simulink model "LPV_ReducedLPV_Simulation_16b"  (R2016b)
settings: Solver=FixedStepAuto  StartTime=0.0  StopTime=10  FixedStep=ts  RelTol=1e-3
values from neighbouring files (symbols this model uses):
  Im = (1/m)*ones(m,m)    [KPCA_Gaussian.m]    (also in KPCA_Polynomial.m)
  ITest = (1/m)*ones(1,m)    [Reduced_LPV_System.m]
  Kernel_Var = 100    [KPCA_Gaussian.m]    (also in KPCA_Polynomial.m = 2)
  KernelMatrix = zeros(m,m)    [KPCA_Gaussian.m]    (also in KPCA_Polynomial.m)
  KTest = zeros(1,m)    [Reduced_LPV_System.m]
  l = 5    [KPCA_Gaussian.m]    (also in KPCA_Polynomial.m; Plot_Accuracy_Gaussian.m = 6; Plot_Accuracy_PCA_Polynomial.m = 6; Plot_Accuracy_Polynomial.m = 6)
  m = 7000    [KPCA_Gaussian.m]    (also in KPCA_Polynomial.m; Plot_Accuracy_Gaussian.m; Plot_Accuracy_PCA_Polynomial.m; Plot_Accuracy_Polynomial.m)
  SortedEigVec = EigVec(:,index)    [KPCA_Gaussian.m]    (also in KPCA_Polynomial.m)
  Training_Data = Param(1:m,:)    [KPCA_Gaussian.m]    (also in KPCA_Polynomial.m)
  ts = 0.01    [InitGyro.m]    (also in Parameters.m)
libraries: simulink x2, cstblocks x2
settings Model: Creator=c00rts28  LastModifiedBy=c00rts28

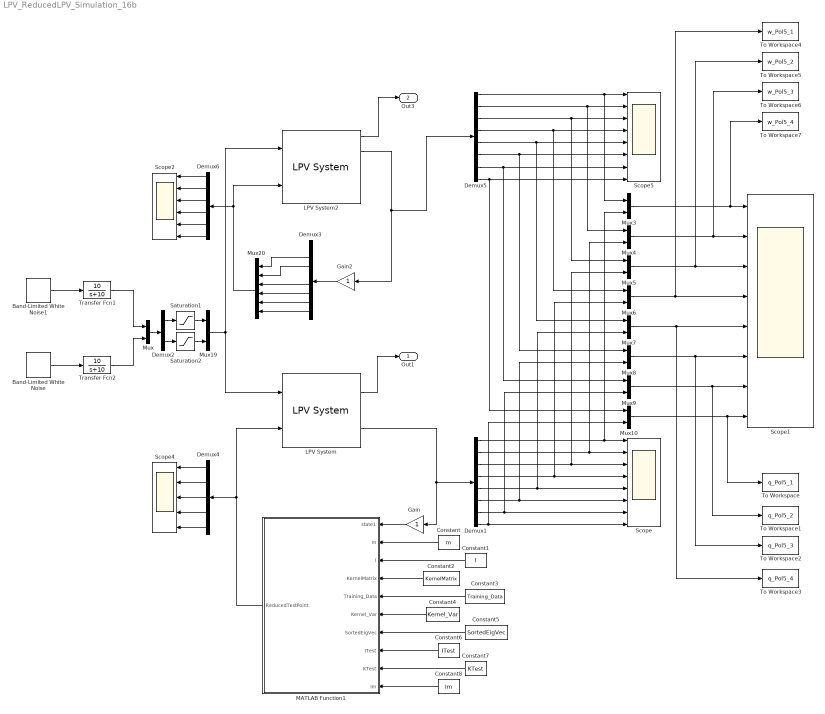
== system LPV_ReducedLPV_Simulation_16b ==
  Band-Limited White Noise : simulink/Sources/Band-Limited White Noise  Cov=[0.000000001]  Ts=ts  seed=[23341]
  Band-Limited White Noise1 : simulink/Sources/Band-Limited White Noise  Cov=[0.000000001]  Ts=ts  seed=[23341]
  Constant : Constant  Value=m
  Constant1 : Constant  Value=l
  Constant2 : Constant  Value=KernelMatrix
  Constant3 : Constant  Value=Training_Data
  Constant4 : Constant  Value=Kernel_Var
  Constant5 : Constant  Value=SortedEigVec
  Constant6 : Constant  Value=ITest
  Constant7 : Constant  Value=KTest
  Constant8 : Constant  Value=Im
  Demux1 : Demux  Outputs=8
  Demux2 : Demux  Outputs=2
  Demux3 : Demux  Outputs=8
  Demux4 : Demux  Outputs=5
  Demux5 : Demux  Outputs=8
  Demux6 : Demux  Outputs=6
  Gain : Gain
  Gain2 : Gain
  LPV System : cstblocks/LPV System  sys=sysReduced  x0=[0.9 0.2 0.1 0.2 0.8 0.4 0.3 0.4]';  uOffset=0  yOffset=0  xOffset=0  opEquilOption=on  dxOffset=0  sysFixedOption=Use the first model in state-space array  sysFixed=[]  AFixed=0  BFixed=0  CFixed=0  DFixed=0  uDelayFixed=true  yDelayFixed=true  iDelayFixed=true  IMethod=Linear  EMethod=Clip  IndexSearch=Binary search  IndexBegin=on  OutputX=on  OutputXdot=off  OutputLTI=off  OutputOP=off  DataType=double  SimMode=Interpreted execution  InitBufferSize=1024  FixedBuffer=off
  LPV System2 : cstblocks/LPV System  sys=sysLPV  x0=[0.9 0.2 0.1 0.2 0.8 0.4 0.3 0.4]';  uOffset=0  yOffset=0  xOffset=0  opEquilOption=off  dxOffset=0  sysFixedOption=Use the first model in state-space array  sysFixed=[]  AFixed=0  BFixed=0  CFixed=0  DFixed=0  uDelayFixed=true  yDelayFixed=true  iDelayFixed=true  IMethod=Linear  EMethod=Clip  IndexSearch=Binary search  IndexBegin=on  OutputX=on  OutputXdot=on  OutputLTI=on  OutputOP=on  DataType=double  SimMode=Interpreted execution  InitBufferSize=1024  FixedBuffer=off
  MATLAB Function1 : MATLAB Function  TreatAsAtomicUnit=on
  Mux{,3..10,19} (10 alike) : Mux  Inputs=2
  Mux20 : Mux  Inputs=6
  Saturation1 : Saturate  UpperLimit=0.666  LowerLimit=-0.666
  Saturation2 : Saturate  UpperLimit=2.44  LowerLimit=-2.44
  Scope : Scope  NumInputPorts=8
  Scope1 : Scope  NumInputPorts=8
  Scope2 : Scope  NumInputPorts=6
  Scope4 : Scope  NumInputPorts=5
  Scope5 : Scope  NumInputPorts=8
  To Workspace : ToWorkspace  VariableName=q_Pol5_1  SaveFormat=Timeseries  SampleTime=-1
  To Workspace1 : ToWorkspace  VariableName=q_Pol5_2  SaveFormat=Timeseries  SampleTime=-1
  To Workspace2 : ToWorkspace  VariableName=q_Pol5_3  SaveFormat=Timeseries  SampleTime=-1
  To Workspace3 : ToWorkspace  VariableName=q_Pol5_4  SaveFormat=Timeseries  SampleTime=-1
  To Workspace4 : ToWorkspace  VariableName=w_Pol5_1  SaveFormat=Timeseries  SampleTime=-1
  To Workspace5 : ToWorkspace  VariableName=w_Pol5_2  SaveFormat=Timeseries  SampleTime=-1
  To Workspace6 : ToWorkspace  VariableName=w_Pol5_3  SaveFormat=Timeseries  SampleTime=-1
  To Workspace7 : ToWorkspace  VariableName=w_Pol5_4  SaveFormat=Timeseries  SampleTime=-1
  Transfer Fcn1 : TransferFcn  Numerator=[10]  Denominator=[1 10]
  Transfer Fcn2 : TransferFcn  Numerator=[10]  Denominator=[1 10]
  Out1 : Outport
  Out3 : Outport  Port=2
  wires:
  LPV System/2 -> Demux1/1, Gain/1
  Gain/1 -> MATLAB Function1/1(state1)
  Constant/1 -> MATLAB Function1/2(m)
  Constant1/1 -> MATLAB Function1/3(l)
  Constant2/1 -> MATLAB Function1/4(KernelMatrix)
  Constant3/1 -> MATLAB Function1/5(Training_Data)
  Constant4/1 -> MATLAB Function1/6(Kernel_Var)
  Constant5/1 -> MATLAB Function1/7(SortedEigVec)
  MATLAB Function1/1(ReducedTestPoint) -> LPV System/2, Demux4/1
  Constant6/1 -> MATLAB Function1/8(ITest)
  Constant7/1 -> MATLAB Function1/9(KTest)
  Constant8/1 -> MATLAB Function1/10(Im)
  Demux1/1 -> Scope/1, Mux3/2
  Demux1/2 -> Scope/2, Mux4/2
  Demux1/3 -> Scope/3, Mux5/2
  Demux1/4 -> Scope/4, Mux6/2
  Demux1/5 -> Scope/5, Mux7/2
  Demux1/6 -> Scope/6, Mux8/2
  Demux1/7 -> Scope/7, Mux9/2
  Demux1/8 -> Scope/8, Mux10/2
  Mux3/1 -> To Workspace7/1, Scope1/1
  Mux5/1 -> To Workspace5/1, Scope1/3
  Mux6/1 -> To Workspace4/1, Scope1/4
  Mux8/1 -> To Workspace2/1, Scope1/6
  Mux9/1 -> To Workspace1/1, Scope1/7
  Mux10/1 -> To Workspace/1, Scope1/8
  Mux20/1 -> Demux6/1, LPV System2/2
  Demux2/1 -> Saturation1/1
  Saturation1/1 -> Mux19/1
  Saturation2/1 -> Mux19/2
  Demux2/2 -> Saturation2/1
  Mux19/1 -> LPV System/1, LPV System2/1
  LPV System2/2 -> Demux5/1, Gain2/1
  Gain2/1 -> Demux3/1
  Demux3/8 -> Mux20/6
  Demux3/7 -> Mux20/5
  Demux3/6 -> Mux20/4
  Demux3/5 -> Mux20/3
  Demux3/2 -> Mux20/1
  Demux3/3 -> Mux20/2
  Mux/1 -> Demux2/1
  Demux5/1 -> Scope5/1, Mux3/1
  Demux5/2 -> Scope5/2, Mux4/1
  Demux5/3 -> Scope5/3, Mux5/1
  Demux5/4 -> Scope5/4, Mux6/1
  Demux5/5 -> Scope5/5, Mux7/1
  Demux5/6 -> Scope5/6, Mux8/1
  Demux5/7 -> Scope5/7, Mux9/1
  Demux5/8 -> Scope5/8, Mux10/1
  LPV System2/1 -> Out3/1
  LPV System/1 -> Out1/1
  Demux4/1 -> Scope4/1
  Demux6/1 -> Scope2/1
  Demux6/2 -> Scope2/2
  Demux6/3 -> Scope2/3
  Demux6/4 -> Scope2/4
  Demux6/5 -> Scope2/5
  Demux6/6 -> Scope2/6
  Mux4/1 -> To Workspace6/1, Scope1/2
  Mux7/1 -> To Workspace3/1, Scope1/5
  Transfer Fcn1/1 -> Mux/1
  Transfer Fcn2/1 -> Mux/2
  Band-Limited White Noise1/1 -> Transfer Fcn1/1
  Band-Limited White Noise/1 -> Transfer Fcn2/1
  Demux4/2 -> Scope4/2
  Demux4/3 -> Scope4/3
  Demux4/5 -> Scope4/5
  Demux4/4 -> Scope4/4

== matlab function LPV_ReducedLPV_Simulation_16b/MATLAB Function1 ==
  data: state1 input size=[8,1]; ReducedTestPoint output double size=[1,5]; m input size=1; l input size=1; KernelMatrix input size=[7000,7000]; Training_Data input size=[7000,6]; Kernel_Var input size=1; SortedEigVec input size=[7000,7000]; ITest input size=[1,7000]; KTest input size=[1,7000]; Im input size=[7000,7000]
function ReducedTestPoint = fcn(state1,m,l,KernelMatrix,Training_Data,Kernel_Var,SortedEigVec,ITest,KTest,Im)

TestPoint = [state1(2) state1(3) state1(5) state1(6) state1(7) state1(8)];


%% Projection of Test Points on first l Eigenvectors
%extract features from the first l Eigenvectors
%Step 1: Choose the kernel function Gaussian or polynomial the same as in 
%the step of training KPCA algoritm 
%step 2: While running the simulation it calculates the new Kernel Matrix KTest
%using test Points And training Examples
%Step 3: Using the trained eigenvectors found from original kernel matrix,
%reduce the dimention of test points
%Note: According to the number of training data points and number of reduced 
%parameters you need to specify the dimension of variables in this 
%matlab function. you can do it from the link "edit data" above. 
%%%%%%%%%%%%%%%%%%%%%%%%%%%%%%%%%%%%%%%%%%%%%%%%%%%%%%%%%%%%%%%%%%%%%%%%%%%

%Polynomial kernel
for j=1:m
    KTest(1,j) = KTest(1,j) + (TestPoint*(Training_Data(j,:)'))^(Kernel_Var);   
end
KTest_Centered = KTest - (ITest*KernelMatrix) - (KTest*Im) + (ITest*KernelMatrix*Im);

%Gaussian kernel
%for j=1:m
%    KTest(1,j) = KTest(1,j) + exp(-(norm(TestPoint-Training_Data(j,:))^2)/Kernel_Var);
%end
%KTest_Centered = KTest - (ITest*KernelMatrix) - (KTest*Im) + (ITest*KernelMatrix*Im);

%we have chosen l to be equal to 5. change it according to the desired
%number of reduced parameters
%%%%%%%%%%%%%%%%%%%%%%%%%%%%%%%%%%%%%%%%%%%%%%%%%%%%%%%%%%%%%%%%%%%%%%%
ReducedTestPoint = real(KTest_Centered*SortedEigVec(:,1:5));

end
